simulink subsystem "GenericWinCmd"  (R2022b)
settings: Solver=VariableStepAuto  StartTime=0.0  StopTime=10.0  RelTol=1e-3
model mask{msgs=0}
  mask prompts: msgs "Messages"
libraries: simulink x1
settings Model: Creator=BEATOA  LastModifiedBy=BEATOA

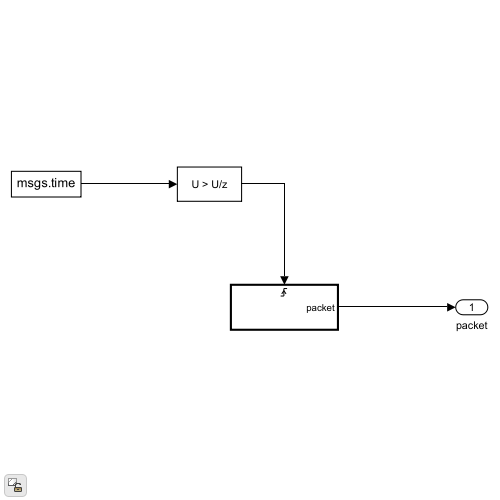
[thumbnail: Simulink's stored preview of the top-level diagram]
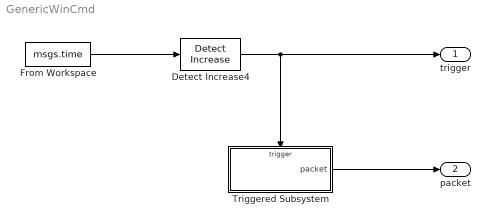
== system GenericWinCmd ==
  Detect Increase4 : simulink/Logic and Bit Operations/Detect Increase  vinit=0.0  OutDataTypeStr=boolean
  From Workspace : FromWorkspace  VariableName=msgs.time  Interpolate=off  OutputAfterFinalValue=Holding final value
  Triggered Subsystem : Subsystem  TreatAsAtomicUnit=on
  trigger : Outport
  packet : Outport  Port=2
  wires:
  From Workspace/1 -> Detect Increase4/1
  Detect Increase4/1 -> Triggered Subsystem/Trigger, trigger/1
  Triggered Subsystem/1(packet) -> packet/1

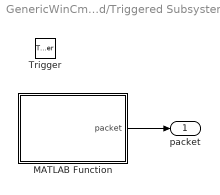
== system GenericWinCmd/Triggered Subsystem ==
  Trigger : TriggerPort  VariantControl=(inherit)
  MATLAB Function : MATLAB Function  TreatAsAtomicUnit=on  mask{msgs=msgs.packets}
      mask prompts: msgs "Packets"
  packet : Outport
  wires:
  MATLAB Function/1(packet) -> packet/1

== matlab function GenericWinCmd/Triggered Subsystem/MATLAB Function ==
  data: packet output; msgs parameter
function packet  = generic_gen(msgs)
persistent index
if isempty(index)
    index = 1;
end
packet = msgs(index,:)';
index = index + 1;
